simulink model "sampleModel5_EMI_Var"  (R2017a)
settings: Solver=VariableStepAuto  StartTime=0.0  StopTime=10.0  RelTol=1e-3
undefined symbols (not defined in the file or in its folder): DiscIntNeverNeededParam
libraries: simulink x32
settings Model: Creator=cyfuzz  LastModifiedBy=cyfuzz

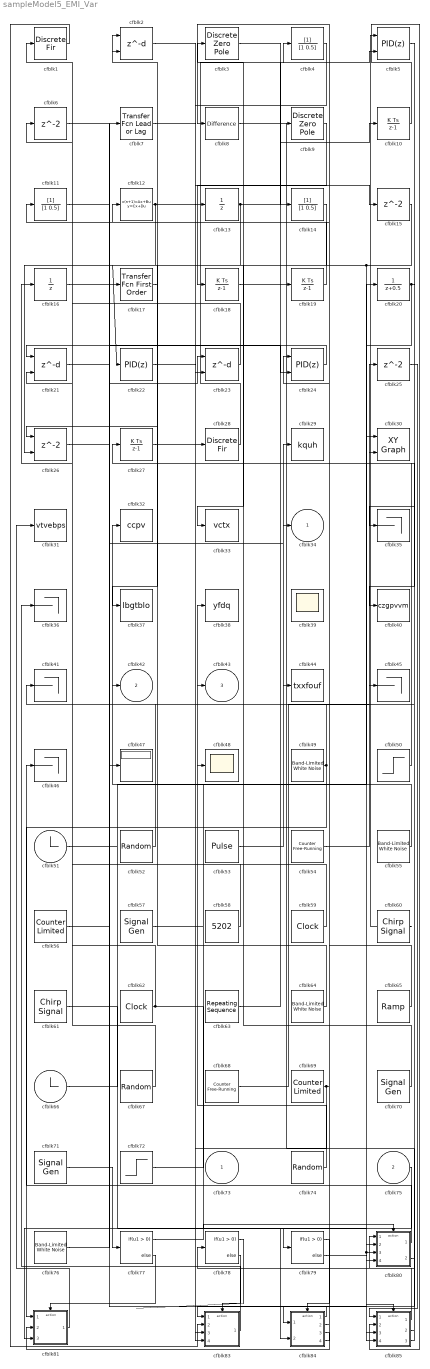
== system sampleModel5_EMI_Var ==
  cfblk73 : Inport
  cfblk75 : Inport  Port=2
  cfblk1 : DiscreteFir  SampleTime=1
  cfblk{10,18..19,27} (4 alike) : DiscreteIntegrator  InitialConditionSetting=State (most efficient)  ICPrevOutput=DiscIntNeverNeededParam  ICPrevScaledInput=DiscIntNeverNeededParam
  cfblk11 : DiscreteFilter  SampleTime=1
  cfblk12 : DiscreteStateSpace
  cfblk13 : UnitDelay
  cfblk14 : DiscreteFilter  SampleTime=1
  cfblk15 : Delay  SampleTime=1
  cfblk16 : UnitDelay
  cfblk17 : simulink/Discrete/Transfer Fcn First Order  PoleZ=0.95  ICPrevOutput=0.0  DoSatur=off
      settings: SourceProductName=Simulink
  cfblk2 : Delay  DelayLengthSource=Input port  SampleTime=1
      settings: InputPortMap=u0,p1
  cfblk20 : DiscreteTransferFcn  SampleTime=1
  cfblk21 : Delay  DelayLengthSource=Input port  SampleTime=1
      settings: InputPortMap=u0,p1
  cfblk22 : simulink/Continuous/PID Controller  Controller=PID  TimeDomain=Discrete-time  SampleTime=1  IntegratorMethod=Forward Euler  FilterMethod=Forward Euler  Form=Parallel  UseFilter=on  ControllerParametersSource=internal  P=1  I=1  D=0  N=100  InitialConditionSource=internal  InitialConditionForIntegrator=0  InitialConditionForFilter=0  ExternalReset=none  LimitOutput=off  UpperSaturationLimit=inf  LowerSaturationLimit=-inf  LinearizeAsGain=off  AntiWindupMode=none  Kb=1  TrackingMode=off  Kt=1  PParamMin=[]  PParamMax=[]  IParamMin=[]  IParamMax=[]  DParamMin=[]  DParamMax=[]  NParamMin=[]  NParamMax=[]  KbParamMin=[]  KbParamMax=[]  KtParamMin=[]  KtParamMax=[]  POutMin=[]  POutMax=[]  IOutMin=[]  IOutMax=[]  DOutMin=[]  DOutMax=[]  NOutMin=[]  NOutMax=[]  KbOutMin=[]  KbOutMax=[]  KtOutMin=[]  KtOutMax=[]  IntegratorOutMin=[]  IntegratorOutMax=[]  FilterOutMin=[]  FilterOutMax=[]  SumOutMin=[]  SumOutMax=[]  SumI1OutMin=[]  SumI1OutMax=[]  SumI2OutMin=[]  SumI2OutMax=[]  SumI3OutMin=[]  SumI3OutMax=[]  SumDOutMin=[]  SumDOutMax=[]  SaturationOutMin=[]  SaturationOutMax=[]  IntegratorContinuousStateAttributes=''  IntegratorStateMustResolveToSignalObject=off  IntegratorRTWStateStorageClass=Auto  FilterContinuousStateAttributes=''  FilterStateMustResolveToSignalObject=off  FilterRTWStateStorageClass=Auto  DifferentiatorICPrevScaledInput=0  DifferentiatorOutMin=[]  DifferentiatorOutMax=[]  InitialConditionSetting=State (most efficient)
  cfblk23 : Delay  DelayLengthSource=Input port  SampleTime=1
      settings: InputPortMap=u0,p1
  cfblk24 : simulink/Continuous/PID Controller (2DOF)  Controller=PID  TimeDomain=Discrete-time  SampleTime=1  IntegratorMethod=Forward Euler  FilterMethod=Forward Euler  Form=Parallel  UseFilter=on  ControllerParametersSource=internal  P=1  I=1  D=0  N=100  b=1  c=1  InitialConditionSource=internal  InitialConditionForIntegrator=0  InitialConditionForFilter=0  ExternalReset=none  LimitOutput=off  UpperSaturationLimit=inf  LowerSaturationLimit=-inf  LinearizeAsGain=off  AntiWindupMode=none  Kb=1  TrackingMode=off  Kt=1  PParamMin=[]  PParamMax=[]  IParamMin=[]  IParamMax=[]  DParamMin=[]  DParamMax=[]  NParamMin=[]  NParamMax=[]  bParamMin=[]  bParamMax=[]  cParamMin=[]  cParamMax=[]  KbParamMin=[]  KbParamMax=[]  KtParamMin=[]  KtParamMax=[]  POutMin=[]  POutMax=[]  IOutMin=[]  IOutMax=[]  DOutMin=[]  DOutMax=[]  NOutMin=[]  NOutMax=[]  bOutMin=[]  bOutMax=[]  cOutMin=[]  cOutMax=[]  KbOutMin=[]  KbOutMax=[]  KtOutMin=[]  KtOutMax=[]  IntegratorOutMin=[]  IntegratorOutMax=[]  FilterOutMin=[]  FilterOutMax=[]  SumOutMin=[]  SumOutMax=[]  Sum1OutMin=[]  Sum1OutMax=[]  Sum2OutMin=[]  Sum2OutMax=[]  Sum3OutMin=[]  Sum3OutMax=[]  SumI1OutMin=[]  SumI1OutMax=[]  SumI2OutMin=[]  SumI2OutMax=[]  SumI3OutMin=[]  SumI3OutMax=[]  SumDOutMin=[]  SumDOutMax=[]  SaturationOutMin=[]  SaturationOutMax=[]  IntegratorContinuousStateAttributes=''  IntegratorStateMustResolveToSignalObject=off  IntegratorRTWStateStorageClass=Auto  FilterContinuousStateAttributes=''  FilterStateMustResolveToSignalObject=off  FilterRTWStateStorageClass=Auto  DifferentiatorICPrevScaledInput=0  DifferentiatorOutMin=[]  DifferentiatorOutMax=[]  InitialConditionSetting=State (most efficient)
  cfblk25 : Delay  SampleTime=1
  cfblk26 : Delay  ShowEnablePort=on  SampleTime=1
      settings: InputPortMap=u0,e6
  cfblk28 : DiscreteFir  SampleTime=1
  cfblk29 : ToFile  Filename=kquh  SaveFormat=Timeseries
  cfblk3 : DiscreteZeroPole  Poles=[0 0.5]  Gain=1
  cfblk30 : simulink/Sinks/XY Graph  xmin=-1  xmax=1  ymin=-1  ymax=1  st=-1
  cfblk31 : ToWorkspace  VariableName=vtvebps  SaveFormat=Timeseries  SampleTime=-1
  cfblk32 : ToFile  Filename=ccpv  SaveFormat=Timeseries
  cfblk33 : ToFile  Filename=vctx  SaveFormat=Timeseries
  cfblk{35..36,41,45..46} (5 alike) : Terminator
  cfblk37 : ToWorkspace  VariableName=lbgtblo  SaveFormat=Timeseries  SampleTime=-1
  cfblk38 : ToFile  Filename=yfdq  SaveFormat=Timeseries
  cfblk39 : Scope
      settings: Floating=on
  cfblk4 : DiscreteFilter  SampleTime=1
  cfblk40 : ToWorkspace  VariableName=czgpvvm  SaveFormat=Timeseries  SampleTime=-1
  cfblk44 : ToWorkspace  VariableName=txxfouf  SaveFormat=Timeseries  SampleTime=-1
  cfblk47 : Display
  cfblk48 : Scope
  cfblk{49,55,64,76} (4 alike) : simulink/Sources/Band-Limited White Noise  Cov=[0.1]  Ts=0.1  seed=[23341]
  cfblk5 : simulink/Continuous/PID Controller (2DOF)  Controller=PID  TimeDomain=Discrete-time  SampleTime=1  IntegratorMethod=Forward Euler  FilterMethod=Forward Euler  Form=Parallel  UseFilter=on  ControllerParametersSource=internal  P=1  I=1  D=0  N=100  b=1  c=1  InitialConditionSource=internal  InitialConditionForIntegrator=0  InitialConditionForFilter=0  ExternalReset=none  LimitOutput=off  UpperSaturationLimit=inf  LowerSaturationLimit=-inf  LinearizeAsGain=off  AntiWindupMode=none  Kb=1  TrackingMode=off  Kt=1  PParamMin=[]  PParamMax=[]  IParamMin=[]  IParamMax=[]  DParamMin=[]  DParamMax=[]  NParamMin=[]  NParamMax=[]  bParamMin=[]  bParamMax=[]  cParamMin=[]  cParamMax=[]  KbParamMin=[]  KbParamMax=[]  KtParamMin=[]  KtParamMax=[]  POutMin=[]  POutMax=[]  IOutMin=[]  IOutMax=[]  DOutMin=[]  DOutMax=[]  NOutMin=[]  NOutMax=[]  bOutMin=[]  bOutMax=[]  cOutMin=[]  cOutMax=[]  KbOutMin=[]  KbOutMax=[]  KtOutMin=[]  KtOutMax=[]  IntegratorOutMin=[]  IntegratorOutMax=[]  FilterOutMin=[]  FilterOutMax=[]  SumOutMin=[]  SumOutMax=[]  Sum1OutMin=[]  Sum1OutMax=[]  Sum2OutMin=[]  Sum2OutMax=[]  Sum3OutMin=[]  Sum3OutMax=[]  SumI1OutMin=[]  SumI1OutMax=[]  SumI2OutMin=[]  SumI2OutMax=[]  SumI3OutMin=[]  SumI3OutMax=[]  SumDOutMin=[]  SumDOutMax=[]  SaturationOutMin=[]  SaturationOutMax=[]  IntegratorContinuousStateAttributes=''  IntegratorStateMustResolveToSignalObject=off  IntegratorRTWStateStorageClass=Auto  FilterContinuousStateAttributes=''  FilterStateMustResolveToSignalObject=off  FilterRTWStateStorageClass=Auto  DifferentiatorICPrevScaledInput=0  DifferentiatorOutMin=[]  DifferentiatorOutMax=[]  InitialConditionSetting=State (most efficient)
  cfblk50 : Step  After=75  SampleTime=0
  cfblk51 : Clock
  cfblk52 : UniformRandomNumber  SampleTime=0.1
  cfblk53 : DiscretePulseGenerator  PulseType=Time based  Period=10  PulseWidth=5
  cfblk54 : simulink/Sources/Counter Free-Running  NumBits=16  tsamp=-1
  cfblk56 : simulink/Sources/Counter Limited  uplimit=7  tsamp=-1
  cfblk57 : SignalGenerator  Units=rad/sec
  cfblk58 : Constant  Value=5202
  cfblk59 : DigitalClock
  cfblk6 : Delay  SampleTime=1
  cfblk60 : simulink/Sources/Chirp Signal  f1=0.1  T=100  f2=1
  cfblk61 : simulink/Sources/Chirp Signal  f1=0.1  T=100  f2=1
  cfblk62 : DigitalClock
  cfblk63 : simulink/Sources/Repeating Sequence  rep_seq_t=[0 2]  rep_seq_y=[0 2]
  cfblk65 : simulink/Sources/Ramp  slope=1  start=0  X0=0
  cfblk66 : Clock
  cfblk67 : RandomNumber  SampleTime=0.1
  cfblk68 : simulink/Sources/Counter Free-Running  NumBits=16  tsamp=-1
  cfblk69 : simulink/Sources/Counter Limited  uplimit=7  tsamp=-1
  cfblk7 : simulink/Discrete/Transfer Fcn Lead or Lag  PoleZ=0.95  ZeroZ=0.75  ICPrevOutput=0.0  ICPrevInput=0.0  DoSatur=off
      settings: SourceProductName=Simulink  SourceProductBaseCode=SL
  cfblk70 : SignalGenerator  Units=rad/sec
  cfblk71 : SignalGenerator  Units=rad/sec
  cfblk72 : Step  After=95  SampleTime=0
  cfblk74 : RandomNumber  SampleTime=0.1
  cfblk77 : If  SampleTime=1
  cfblk78 : If  SampleTime=1
  cfblk79 : If  SampleTime=1
  cfblk8 : simulink/Discrete/Difference  ICPrevInput=0.0  OutMin=[]  OutMax=[]  OutDataTypeStr=Inherit: Inherit via back propagation  OutDataType=fixdt(1, 16)  OutScaling=2^-10  DoSatur=off
  cfblk80 : Subsystem  TreatAsAtomicUnit=on
  cfblk81 : Subsystem  TreatAsAtomicUnit=on
  cfblk83 : Subsystem  TreatAsAtomicUnit=on
  cfblk84 : Subsystem  TreatAsAtomicUnit=on
  cfblk85 : Subsystem  TreatAsAtomicUnit=on
  cfblk9 : DiscreteZeroPole  Poles=[0 0.5]  Gain=1
  cfblk34 : Outport
  cfblk42 : Outport  Port=2
  cfblk43 : Outport  Port=3
  wires:
  cfblk80/1(cfblk2) -> cfblk46/1
  cfblk8/1 -> cfblk84/1(cfblk1)
  cfblk72/1 -> cfblk29/1
  cfblk83/1(cfblk2) -> cfblk36/1
  cfblk84/1(cfblk2) -> cfblk83/1(cfblk1)
  cfblk28/1 -> cfblk4/1
  cfblk9/1 -> cfblk18/1
  cfblk69/1 -> cfblk8/1, cfblk83/4(cfblk12)
  cfblk81/1(cfblk2) -> cfblk31/1
  cfblk25/1 -> cfblk85/1(cfblk1)
  cfblk15/1 -> cfblk22/1, cfblk80/4(cfblk8)
  cfblk17/1 -> cfblk26/1
  cfblk50/1 -> cfblk27/1
  cfblk7/1 -> cfblk15/1
  cfblk54/1 -> cfblk25/1
  cfblk63/1 -> cfblk19/1
  cfblk27/1 -> cfblk28/1
  cfblk71/1 -> cfblk77/1
  cfblk68/1 -> cfblk45/1
  cfblk55/1 -> cfblk32/1
  cfblk5/1 -> cfblk40/1
  cfblk59/1 -> cfblk12/1
  cfblk67/1 -> cfblk16/1
  cfblk2/1 -> cfblk13/1
  cfblk56/1 -> cfblk17/1
  cfblk62/1 -> cfblk84/2(cfblk12), cfblk21/2
  cfblk53/1 -> cfblk44/1
  cfblk76/1 -> cfblk34/1
  cfblk26/1 -> cfblk23/1
  cfblk66/1 -> cfblk9/1
  cfblk20/1 -> cfblk80/3(cfblk7), cfblk85/4(cfblk8), cfblk35/1
  cfblk6/1 -> cfblk47/1
  cfblk58/1 -> cfblk1/1
  cfblk52/1 -> cfblk42/1
  cfblk14/1 -> cfblk33/1
  cfblk70/1 -> cfblk3/1
  cfblk18/1 -> cfblk10/1
  cfblk51/1 -> cfblk20/1
  cfblk74/1 -> cfblk38/1
  cfblk10/1 -> cfblk85/2(cfblk6)
  cfblk1/1 -> cfblk83/2(cfblk10)
  cfblk3/1 -> cfblk14/1
  cfblk84/2(cfblk13) -> cfblk48/1
  cfblk13/1 -> cfblk37/1, cfblk5/2
  cfblk57/1 -> cfblk30/1
  cfblk21/1 -> cfblk7/1
  cfblk61/1 -> cfblk79/1
  cfblk23/1 -> cfblk6/1
  cfblk65/1 -> cfblk24/1
  cfblk64/1 -> cfblk2/1
  cfblk11/1 -> cfblk83/3(cfblk11)
  cfblk85/1(cfblk2) -> cfblk78/1
  cfblk80/2(cfblk9) -> cfblk41/1
  cfblk24/1 -> cfblk21/1
  cfblk19/1 -> cfblk2/2
  cfblk16/1 -> cfblk24/2
  cfblk49/1 -> cfblk81/1(cfblk1), cfblk43/1
  cfblk84/3(cfblk14) -> cfblk81/2(cfblk8)
  cfblk4/1 -> cfblk23/2
  cfblk85/2(cfblk9) -> cfblk30/2
  cfblk12/1 -> cfblk26/2, cfblk80/2(cfblk6)
  cfblk85/3(cfblk10) -> cfblk80/1(cfblk1)
  cfblk75/1 -> cfblk81/3(cfblk9)
  cfblk84/4(cfblk15) -> cfblk11/1
  cfblk22/1 -> cfblk85/3(cfblk7)
  cfblk77/1 -> cfblk80/Action
  cfblk77/2 -> cfblk81/Action
  cfblk78/1 -> ?
  cfblk78/2 -> cfblk83/Action
  cfblk79/1 -> cfblk84/Action
  cfblk79/2 -> cfblk85/Action
  cfblk60/1 -> cfblk5/1

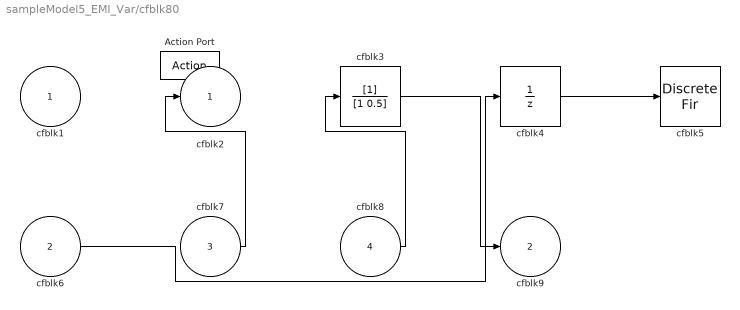
== system sampleModel5_EMI_Var/cfblk80 ==
  cfblk1 : Inport
  cfblk6 : Inport  Port=2
  cfblk7 : Inport  Port=3
  cfblk8 : Inport  Port=4
  Action Port : ActionPort  ActionType=then
  cfblk3 : DiscreteFilter
  cfblk4 : UnitDelay  SampleTime=-1
  cfblk5 : DiscreteFir
  cfblk2 : Outport
  cfblk9 : Outport  Port=2
  wires:
  cfblk7/1 -> cfblk2/1
  cfblk6/1 -> cfblk4/1
  cfblk3/1 -> cfblk9/1
  cfblk8/1 -> cfblk3/1
  cfblk4/1 -> cfblk5/1

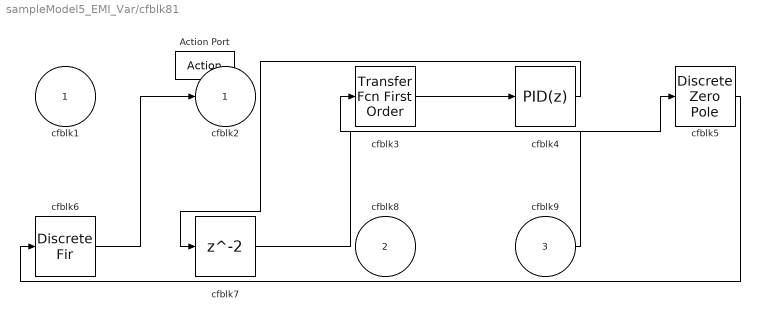
== system sampleModel5_EMI_Var/cfblk81 ==
  cfblk1 : Inport
  cfblk8 : Inport  Port=2
  cfblk9 : Inport  Port=3
  Action Port : ActionPort  ActionType=else
  cfblk3 : simulink/Discrete/Transfer Fcn First Order  PoleZ=0.95  ICPrevOutput=0.0  DoSatur=off
      settings: SourceProductName=Simulink
  cfblk4 : simulink/Continuous/PID Controller  Controller=PID  TimeDomain=Discrete-time  SampleTime=-1  IntegratorMethod=Forward Euler  FilterMethod=Forward Euler  Form=Parallel  UseFilter=on  ControllerParametersSource=internal  P=1  I=1  D=0  N=100  InitialConditionSource=internal  InitialConditionForIntegrator=0  InitialConditionForFilter=0  ExternalReset=none  LimitOutput=off  UpperSaturationLimit=inf  LowerSaturationLimit=-inf  LinearizeAsGain=off  AntiWindupMode=none  Kb=1  TrackingMode=off  Kt=1  PParamMin=[]  PParamMax=[]  IParamMin=[]  IParamMax=[]  DParamMin=[]  DParamMax=[]  NParamMin=[]  NParamMax=[]  KbParamMin=[]  KbParamMax=[]  KtParamMin=[]  KtParamMax=[]  POutMin=[]  POutMax=[]  IOutMin=[]  IOutMax=[]  DOutMin=[]  DOutMax=[]  NOutMin=[]  NOutMax=[]  KbOutMin=[]  KbOutMax=[]  KtOutMin=[]  KtOutMax=[]  IntegratorOutMin=[]  IntegratorOutMax=[]  FilterOutMin=[]  FilterOutMax=[]  SumOutMin=[]  SumOutMax=[]  SumI1OutMin=[]  SumI1OutMax=[]  SumI2OutMin=[]  SumI2OutMax=[]  SumI3OutMin=[]  SumI3OutMax=[]  SumDOutMin=[]  SumDOutMax=[]  SaturationOutMin=[]  SaturationOutMax=[]  IntegratorContinuousStateAttributes=''  IntegratorStateMustResolveToSignalObject=off  IntegratorRTWStateStorageClass=Auto  FilterContinuousStateAttributes=''  FilterStateMustResolveToSignalObject=off  FilterRTWStateStorageClass=Auto  DifferentiatorICPrevScaledInput=0  DifferentiatorOutMin=[]  DifferentiatorOutMax=[]  InitialConditionSetting=State (most efficient)
  cfblk5 : DiscreteZeroPole  Poles=[0 0.5]  Gain=1  SampleTime=-1
  cfblk6 : DiscreteFir
  cfblk7 : Delay
  cfblk2 : Outport
  wires:
  cfblk7/1 -> cfblk5/1
  cfblk9/1 -> cfblk3/1
  cfblk6/1 -> cfblk2/1
  cfblk3/1 -> cfblk4/1
  cfblk4/1 -> cfblk7/1
  cfblk5/1 -> cfblk6/1

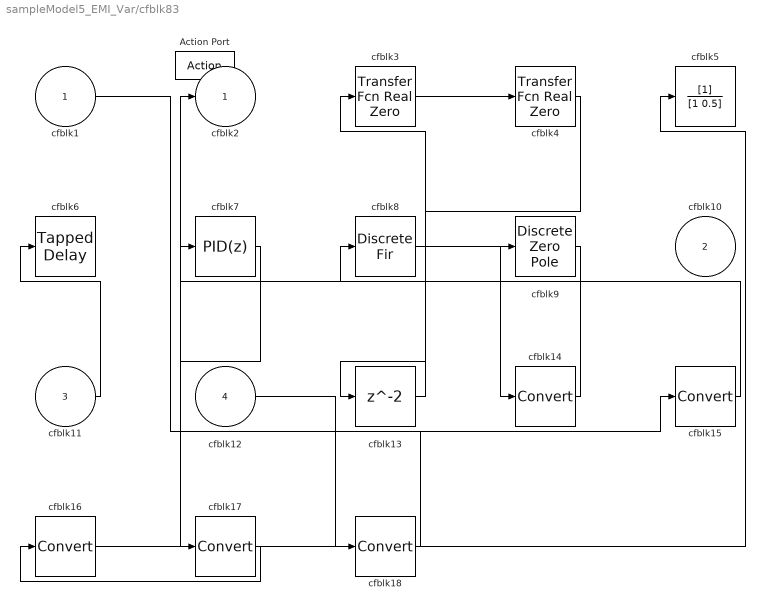
== system sampleModel5_EMI_Var/cfblk83 ==
  cfblk1 : Inport
  cfblk10 : Inport  Port=2
  cfblk11 : Inport  Port=3
  cfblk12 : Inport  Port=4
  Action Port : ActionPort  ActionType=else
  cfblk13 : Delay
  cfblk{14..18} (5 alike) : DataTypeConversion
  cfblk3 : simulink/Discrete/Transfer Fcn Real Zero  ZeroZ=0.75  ICPrevInput=0.0  DoSatur=off
      settings: SourceProductName=Simulink  SourceProductBaseCode=SL
  cfblk4 : simulink/Discrete/Transfer Fcn Real Zero  ZeroZ=0.75  ICPrevInput=0.0  DoSatur=off
      settings: SourceProductName=Simulink  SourceProductBaseCode=SL
  cfblk5 : DiscreteFilter
  cfblk6 : simulink/Discrete/Tapped Delay  vinit=0.0  samptime=-1  NumDelays=1  DelayOrder=Oldest  includeCurrent=off
  cfblk7 : simulink/Continuous/PID Controller  Controller=PID  TimeDomain=Discrete-time  SampleTime=-1  IntegratorMethod=Forward Euler  FilterMethod=Forward Euler  Form=Parallel  UseFilter=on  ControllerParametersSource=internal  P=1  I=1  D=0  N=100  InitialConditionSource=internal  InitialConditionForIntegrator=0  InitialConditionForFilter=0  ExternalReset=none  LimitOutput=off  UpperSaturationLimit=inf  LowerSaturationLimit=-inf  LinearizeAsGain=off  AntiWindupMode=none  Kb=1  TrackingMode=off  Kt=1  PParamMin=[]  PParamMax=[]  IParamMin=[]  IParamMax=[]  DParamMin=[]  DParamMax=[]  NParamMin=[]  NParamMax=[]  KbParamMin=[]  KbParamMax=[]  KtParamMin=[]  KtParamMax=[]  POutMin=[]  POutMax=[]  IOutMin=[]  IOutMax=[]  DOutMin=[]  DOutMax=[]  NOutMin=[]  NOutMax=[]  KbOutMin=[]  KbOutMax=[]  KtOutMin=[]  KtOutMax=[]  IntegratorOutMin=[]  IntegratorOutMax=[]  FilterOutMin=[]  FilterOutMax=[]  SumOutMin=[]  SumOutMax=[]  SumI1OutMin=[]  SumI1OutMax=[]  SumI2OutMin=[]  SumI2OutMax=[]  SumI3OutMin=[]  SumI3OutMax=[]  SumDOutMin=[]  SumDOutMax=[]  SaturationOutMin=[]  SaturationOutMax=[]  IntegratorContinuousStateAttributes=''  IntegratorStateMustResolveToSignalObject=off  IntegratorRTWStateStorageClass=Auto  FilterContinuousStateAttributes=''  FilterStateMustResolveToSignalObject=off  FilterRTWStateStorageClass=Auto  DifferentiatorICPrevScaledInput=0  DifferentiatorOutMin=[]  DifferentiatorOutMax=[]  InitialConditionSetting=State (most efficient)
  cfblk8 : DiscreteFir
  cfblk9 : DiscreteZeroPole  Poles=[0 0.5]  Gain=1  SampleTime=-1
  cfblk2 : Outport
  wires:
  cfblk11/1 -> cfblk6/1
  cfblk9/1 -> cfblk2/1
  cfblk3/1 -> cfblk4/1
  cfblk4/1 -> cfblk13/1
  cfblk13/1 -> cfblk3/1
  cfblk8/1 -> cfblk14/1
  cfblk14/1 -> cfblk9/1
  cfblk1/1 -> cfblk15/1
  cfblk15/1 -> cfblk8/1
  cfblk16/1 -> cfblk5/1
  cfblk7/1 -> cfblk17/1
  cfblk17/1 -> cfblk16/1
  cfblk12/1 -> cfblk18/1
  cfblk18/1 -> cfblk7/1

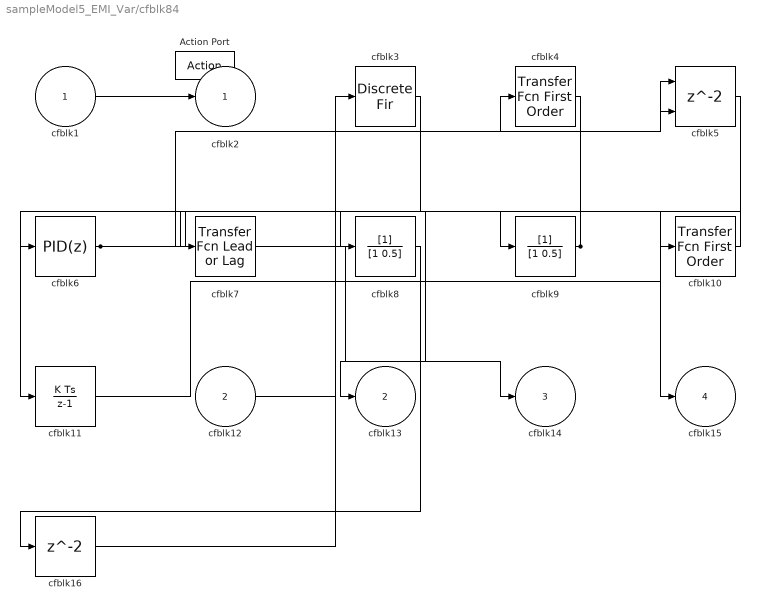
== system sampleModel5_EMI_Var/cfblk84 ==
  cfblk1 : Inport
  cfblk12 : Inport  Port=2
  Action Port : ActionPort  ActionType=then
  cfblk10 : simulink/Discrete/Transfer Fcn First Order  PoleZ=0.95  ICPrevOutput=0.0  DoSatur=off
      settings: SourceProductName=Simulink
  cfblk11 : DiscreteIntegrator  InitialConditionSetting=State (most efficient)  SampleTime=-1  ICPrevOutput=DiscIntNeverNeededParam  ICPrevScaledInput=DiscIntNeverNeededParam
  cfblk16 : Delay
  cfblk3 : DiscreteFir
  cfblk4 : simulink/Discrete/Transfer Fcn First Order  PoleZ=0.95  ICPrevOutput=0.0  DoSatur=off
      settings: SourceProductName=Simulink
  cfblk5 : Delay  ShowEnablePort=on
      settings: InputPortMap=u0,e6
  cfblk6 : simulink/Continuous/PID Controller  Controller=PID  TimeDomain=Discrete-time  SampleTime=-1  IntegratorMethod=Forward Euler  FilterMethod=Forward Euler  Form=Parallel  UseFilter=on  ControllerParametersSource=internal  P=1  I=1  D=0  N=100  InitialConditionSource=internal  InitialConditionForIntegrator=0  InitialConditionForFilter=0  ExternalReset=none  LimitOutput=off  UpperSaturationLimit=inf  LowerSaturationLimit=-inf  LinearizeAsGain=off  AntiWindupMode=none  Kb=1  TrackingMode=off  Kt=1  PParamMin=[]  PParamMax=[]  IParamMin=[]  IParamMax=[]  DParamMin=[]  DParamMax=[]  NParamMin=[]  NParamMax=[]  KbParamMin=[]  KbParamMax=[]  KtParamMin=[]  KtParamMax=[]  POutMin=[]  POutMax=[]  IOutMin=[]  IOutMax=[]  DOutMin=[]  DOutMax=[]  NOutMin=[]  NOutMax=[]  KbOutMin=[]  KbOutMax=[]  KtOutMin=[]  KtOutMax=[]  IntegratorOutMin=[]  IntegratorOutMax=[]  FilterOutMin=[]  FilterOutMax=[]  SumOutMin=[]  SumOutMax=[]  SumI1OutMin=[]  SumI1OutMax=[]  SumI2OutMin=[]  SumI2OutMax=[]  SumI3OutMin=[]  SumI3OutMax=[]  SumDOutMin=[]  SumDOutMax=[]  SaturationOutMin=[]  SaturationOutMax=[]  IntegratorContinuousStateAttributes=''  IntegratorStateMustResolveToSignalObject=off  IntegratorRTWStateStorageClass=Auto  FilterContinuousStateAttributes=''  FilterStateMustResolveToSignalObject=off  FilterRTWStateStorageClass=Auto  DifferentiatorICPrevScaledInput=0  DifferentiatorOutMin=[]  DifferentiatorOutMax=[]  InitialConditionSetting=State (most efficient)
  cfblk7 : simulink/Discrete/Transfer Fcn Lead or Lag  PoleZ=0.95  ZeroZ=0.75  ICPrevOutput=0.0  ICPrevInput=0.0  DoSatur=off
      settings: SourceProductName=Simulink  SourceProductBaseCode=SL
  cfblk8 : DiscreteFilter
  cfblk9 : DiscreteFilter
  cfblk2 : Outport
  cfblk13 : Outport  Port=2
  cfblk14 : Outport  Port=3
  cfblk15 : Outport  Port=4
  wires:
  cfblk3/1 -> cfblk11/1
  cfblk5/1 -> cfblk15/1
  cfblk1/1 -> cfblk2/1
  cfblk11/1 -> cfblk10/1
  cfblk10/1 -> cfblk9/1
  cfblk7/1 -> cfblk14/1
  cfblk6/1 -> cfblk8/1, cfblk5/1, cfblk5/2
  cfblk4/1 -> cfblk13/1
  cfblk9/1 -> cfblk7/1, cfblk6/1
  cfblk12/1 -> cfblk4/1
  cfblk8/1 -> cfblk16/1
  cfblk16/1 -> cfblk3/1

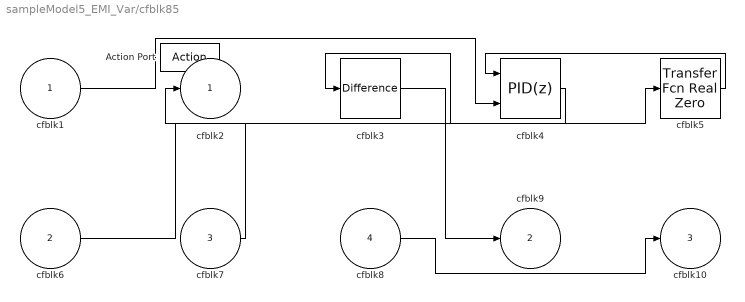
== system sampleModel5_EMI_Var/cfblk85 ==
  cfblk1 : Inport
  cfblk6 : Inport  Port=2
  cfblk7 : Inport  Port=3
  cfblk8 : Inport  Port=4
  Action Port : ActionPort  ActionType=else
  cfblk3 : simulink/Discrete/Difference  ICPrevInput=0.0  OutMin=[]  OutMax=[]  OutDataTypeStr=Inherit: Inherit via back propagation  OutDataType=fixdt(1, 16)  OutScaling=2^-10  DoSatur=off
  cfblk4 : simulink/Continuous/PID Controller (2DOF)  Controller=PID  TimeDomain=Discrete-time  SampleTime=-1  IntegratorMethod=Forward Euler  FilterMethod=Forward Euler  Form=Parallel  UseFilter=on  ControllerParametersSource=internal  P=1  I=1  D=0  N=100  b=1  c=1  InitialConditionSource=internal  InitialConditionForIntegrator=0  InitialConditionForFilter=0  ExternalReset=none  LimitOutput=off  UpperSaturationLimit=inf  LowerSaturationLimit=-inf  LinearizeAsGain=off  AntiWindupMode=none  Kb=1  TrackingMode=off  Kt=1  PParamMin=[]  PParamMax=[]  IParamMin=[]  IParamMax=[]  DParamMin=[]  DParamMax=[]  NParamMin=[]  NParamMax=[]  bParamMin=[]  bParamMax=[]  cParamMin=[]  cParamMax=[]  KbParamMin=[]  KbParamMax=[]  KtParamMin=[]  KtParamMax=[]  POutMin=[]  POutMax=[]  IOutMin=[]  IOutMax=[]  DOutMin=[]  DOutMax=[]  NOutMin=[]  NOutMax=[]  bOutMin=[]  bOutMax=[]  cOutMin=[]  cOutMax=[]  KbOutMin=[]  KbOutMax=[]  KtOutMin=[]  KtOutMax=[]  IntegratorOutMin=[]  IntegratorOutMax=[]  FilterOutMin=[]  FilterOutMax=[]  SumOutMin=[]  SumOutMax=[]  Sum1OutMin=[]  Sum1OutMax=[]  Sum2OutMin=[]  Sum2OutMax=[]  Sum3OutMin=[]  Sum3OutMax=[]  SumI1OutMin=[]  SumI1OutMax=[]  SumI2OutMin=[]  SumI2OutMax=[]  SumI3OutMin=[]  SumI3OutMax=[]  SumDOutMin=[]  SumDOutMax=[]  SaturationOutMin=[]  SaturationOutMax=[]  IntegratorContinuousStateAttributes=''  IntegratorStateMustResolveToSignalObject=off  IntegratorRTWStateStorageClass=Auto  FilterContinuousStateAttributes=''  FilterStateMustResolveToSignalObject=off  FilterRTWStateStorageClass=Auto  DifferentiatorICPrevScaledInput=0  DifferentiatorOutMin=[]  DifferentiatorOutMax=[]  InitialConditionSetting=State (most efficient)
  cfblk5 : simulink/Discrete/Transfer Fcn Real Zero  ZeroZ=0.75  ICPrevInput=0.0  DoSatur=off
      settings: SourceProductName=Simulink  SourceProductBaseCode=SL
  cfblk2 : Outport
  cfblk9 : Outport  Port=2
  cfblk10 : Outport  Port=3
  wires:
  cfblk3/1 -> cfblk9/1
  cfblk5/1 -> cfblk4/1
  cfblk7/1 -> cfblk2/1
  cfblk4/1 -> cfblk3/1
  cfblk1/1 -> cfblk4/2
  cfblk8/1 -> cfblk10/1
  cfblk6/1 -> cfblk5/1
